simulink library "INT_CoTemp"  (R2016b)
settings: Solver=VariableStepAuto  StartTime=0.0  StopTime=10.0  RelTol=1e-3
settings Model: Creator=Administrator  LastModifiedBy=Administrator

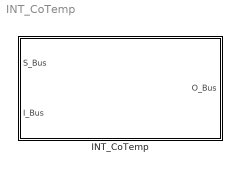
== system INT_CoTemp ==
  INT_CoTemp : Subsystem

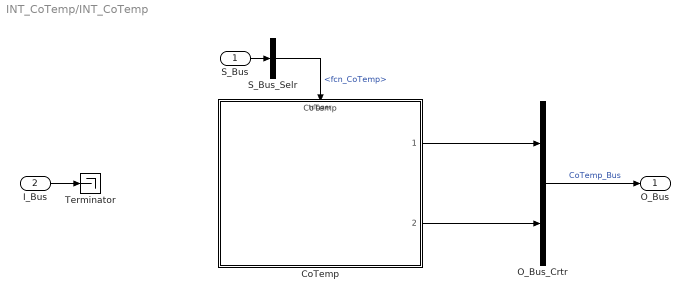
== system INT_CoTemp/INT_CoTemp ==
  S_Bus : Inport
  I_Bus : Inport  Port=2
  CoTemp : ModelReference  ModelNameDialog=CoTemp  SimulationMode=Normal  ModelReferenceVersion=1.2  TriggerPortName=function  TriggerPortTriggerType=function-call  TriggerPortStatesWhenEnabling=held
  O_Bus_Crtr : BusCreator  Inputs=2
  S_Bus_Selr : BusSelector  OutputSignals=fcn_CoTemp
  Terminator : Terminator
  O_Bus : Outport
  wires:
  S_Bus_Selr/1 -> CoTemp/Trigger  "<fcn_CoTemp>"
  S_Bus/1 -> S_Bus_Selr/1
  I_Bus/1 -> Terminator/1
  O_Bus_Crtr/1 -> O_Bus/1  "CoTemp_Bus"
  CoTemp/1 -> O_Bus_Crtr/1
  CoTemp/2 -> O_Bus_Crtr/2
